simulink model "VehCtrlMdel240829_autosar"  (R2019b)
settings: Solver=FixedStepDiscrete  StartTime=0.0  StopTime=10.0  FixedStep=0.0005  RelTol=1e-3  EnableMultiTasking=on
values from neighbouring files (symbols this model uses):
  Ax_OffSet = 0.0    [VehCtrlMdelDictionary.sldd]    (also in VehPara.m = 0)
  Ay_OffSet = 0.0    [VehCtrlMdelDictionary.sldd]    (also in VehPara.m = 0)
  Caf = 460.0    [VehCtrlMdelDictionary.sldd]    (also in VehPara.m = 460; trqvparameter.m = 460)
  Car = 440.0    [VehCtrlMdelDictionary.sldd]    (also in VehPara.m = 440; trqvparameter.m = 440)
  dwf = 1.2    [VehCtrlMdelDictionary.sldd]    (also in VehPara.m; trqvparameter.m)
  Ki = 1.0    [VehCtrlMdelDictionary.sldd]    (also in VehPara.m = 1; trqvparameter.m = 1)
  Kp = 2.0    [VehCtrlMdelDictionary.sldd]    (also in VehPara.m = 2; trqvparameter.m = 2)
  Ldwf = 1.2    [VehCtrlMdelDictionary.sldd]    (also in VehPara.m)
  Ldwr = 1.16    [VehCtrlMdelDictionary.sldd]    (also in VehPara.m)
  lf = 0.761    [VehCtrlMdelDictionary.sldd]    (also in VehPara.m; trqvparameter.m)
  lr = 0.831    [VehCtrlMdelDictionary.sldd]    (also in VehPara.m; trqvparameter.m)
  m = 340.0    [VehCtrlMdelDictionary.sldd]    (also in VehPara.m = 340; trqvparameter.m = 340)
  Offset_Angle = 0.0    [VehCtrlMdelDictionary.sldd]    (also in VehPara.m = 0)
  Qa = 0.1    [VehCtrlMdelDictionary.sldd]    (also in VehPara.m)
  Ra = 2.0    [VehCtrlMdelDictionary.sldd]    (also in VehPara.m = 2)
  RearRatio = 0.8    [VehCtrlMdelDictionary.sldd]    (also in VehPara.m)
  Rt = 0.2    [VehCtrlMdelDictionary.sldd]    (also in VehPara.m; trqvparameter.m)
  thr1 = 2.0    [VehCtrlMdelDictionary.sldd]    (also in VehPara.m = 2)
  thr2 = 0.5    [VehCtrlMdelDictionary.sldd]    (also in VehPara.m)
  thr3 = 0.8    [VehCtrlMdelDictionary.sldd]    (also in VehPara.m)
  thr4 = 0.5    [VehCtrlMdelDictionary.sldd]    (also in VehPara.m)
  thr5 = -0.5    [VehCtrlMdelDictionary.sldd]    (also in VehPara.m)
  TrqRquRate = 0.1    [VehCtrlMdelDictionary.sldd]    (also in VehPara.m)
  YawRate_OffSet = 0.0    [VehCtrlMdelDictionary.sldd]    (also in VehPara.m = 0)
undefined symbols (not defined in the file or in its folder): DiscIntNeverNeededParam, I_AN07_5V, I_AN08_5V, I_AN10_5V, I_SW01_L, I_SW02_L, I_SW03_L, Iz, O_SW12_HS1A, O_SW14_HS1A, PWM3
libraries: simulink x126, ec5744lib x77, canmsglib x18
(part 5 of 5)

== stateflow chart VehCtrlMdel240829_autosar/Drive_Ready/Subsystem/Chart2 ==
  state VehStat [parallel]
    settings: executionOrder=1
    state WaitForEngine
      en:
      send(AMKCANOFF,AMKCANenable);
      send(AMKDCOFF,AMKDCon);
      send(MCDCEnableOFF,MCDCEnable);
      send(InverterOFF,MC_InverterOn);
    state Standby
    state Trans
    state Guard
    state InitStateBack
    state Ready
    state Init
      en:
      errorReset = 1;
    state MCUReadyFail
    WaitForEngine -> Standby : [aMCUReady&&bMCUReady&&cMCUReady]
    Standby -> Guard [order 2] : [KeyPressed&&Brk&&ACC_Release&&cMCUReady&&aMCUReady&&bMCUReady]
    Trans -> Ready : after(2.5,sec){send(EbeepOFF,BeeperStat)}
    Guard -> Trans [order 1] : after(0.25,sec){send(EbeepON,BeeperStat)}
    Guard -> Standby [order 2] : [~KeyPressed||~Brk||~ACC_Release]
    Standby -> WaitForEngine [order 1] : [~aMCUReady||~bMCUReady||~cMCUReady]
    Guard -> InitStateBack [order 3] : [~cMCUReady||~aMCUReady||~bMCUReady]
    Init -> WaitForEngine : [after(1,sec)]
    MCUReadyFail -> WaitForEngine
    InitStateBack -> WaitForEngine
    Ready -> InitStateBack [order 2] : [~HVCutOFF]
    (default) -> Init
    Ready -> MCUReadyFail [order 1] : [~cMCUReady||~aMCUReady||~bMCUReady]
  state BeeperStat [parallel]
    settings: executionOrder=2
    state OFF
    state ON
    (default) -> BeeperStat.OFF
    BeeperStat.OFF -> BeeperStat.ON : EbeepON
    BeeperStat.ON -> BeeperStat.OFF : EbeepOFF
  state AMKDCon [parallel]
    settings: executionOrder=6
    state OFF
    state ON
    (default) -> AMKDCon.OFF
    AMKDCon.OFF -> AMKDCon.ON : AMKDCON
    AMKDCon.ON -> AMKDCon.OFF : AMKDCOFF
  state MCDCEnable [parallel]
    settings: executionOrder=7
    state OFF
    state ON
    (default) -> MCDCEnable.OFF
    MCDCEnable.OFF -> MCDCEnable.ON : MCDCEnableON
    MCDCEnable.ON -> MCDCEnable.OFF : MCDCEnableOFF
  state AMKDCready [parallel]
    settings: executionOrder=4
    state start
    state AMKCAN
      en:
      send(AMKCANON,AMKCANenable);
    state MC_DCready
    state MCDCOncheck
    state DCOnCheckPass
    state MC_DCOnFail
      en:
      send(AMKDCOFF,AMKDCon);
      send(MCDCEnableOFF,MCDCEnable);
      send(InverterOFF,MC_InverterOn);
    state AMKDCOnFinish
    state SYSRDYCECK
    state MCDCEnableState
      en:
      send(MCDCEnableON,MCDCEnable);
    state MC_InverterOn_State
      en:
      send(InverterON,MC_InverterOn);
    (default) -> start
    AMKCAN -> MC_DCready : [SWAMKDCOn]
    MC_DCready -> MCDCOncheck [order 2] : after(0.1,sec){send(AMKDCON,AMKDCon)}
    MCDCOncheck -> DCOnCheckPass [order 1] : after(0.1,sec)
    start -> AMKCAN : after(10,sec)
    DCOnCheckPass -> MCDCEnableState : after(0.1,sec)[MCFLDCOncheck&&MCFRDCOncheck]
    MCDCOncheck -> MC_DCOnFail [order 2] : [~MCFRDCOncheck||~MCFLDCOncheck]
    MC_DCready -> AMKCAN [order 1] : [~SWAMKDCOn]
    SYSRDYCECK -> MC_DCOnFail [order 2] : [~MCFL_SYSREADY||~MCFR_SYSREADY]
    SYSRDYCECK -> AMKDCOnFinish [order 1] : [MCFL_SYSREADY&&MCFR_SYSREADY]
    MC_InverterOn_State -> SYSRDYCECK
    MCDCEnableState -> MC_InverterOn_State : after(0.1,sec)
  state Output [parallel]
    du:
    VehReady = in(VehStat.Ready);
    VehStandby = in(VehStat.Standby);
    BeeperStOut = in(BeeperStat.ON);
    AMKCANready = in(AMKCANenable.ON);
    MCFL_DCOn_setpoints = in(AMKDCon.ON);
    MCFR_DCOn_setpoints = in(AMKDCon.ON);
    MCFL_DCEnable = in(MCDCEnable.ON);
    MCFR_DCEnable = in(MCDCEnable.ON);
    MC_DCOnError = in(AMKDCready.MC_DCOnFail);
    MCFL_InverterOn = in(MC_InverterOn.ON);
    MCFR_InverterOn = in(MC_InverterOn.ON);
    settings: executionOrder=3
  state AMKCANenable [parallel]
    settings: executionOrder=5
    state OFF
    state ON
    (default) -> AMKCANenable.OFF
    AMKCANenable.OFF -> AMKCANenable.ON : AMKCANON
    AMKCANenable.ON -> AMKCANenable.OFF : AMKCANOFF
  state MC_InverterOn [parallel]
    settings: executionOrder=8
    state OFF
    state ON
    (default) -> MC_InverterOn.OFF
    MC_InverterOn.OFF -> MC_InverterOn.ON : InverterON
    MC_InverterOn.ON -> MC_InverterOn.OFF : InverterOFF
  data: Brk input boolean size=1; KeyPressed input boolean size=1; VehReady output boolean size=1; BeeperStOut output boolean size=1; VehStandby output boolean; ACC_Release input boolean; cMCUReady input; aMCUReady input; bMCUReady input; AMKCANready output; MCFL_DCOn_setpoints output; MCFRDCOncheck input; MCFLDCOncheck input; MCFR_DCOn_setpoints output; MCFR_DCEnable output; MCFR_InverterOn output; MC_DCOnError output; MCFL_InverterOn output; MCFL_DCEnable output; MCFL_SYSREADY input; MCFR_SYSREADY input; SWAMKDCOn input; HVCutOFF input; errorReset output
  events: EbeepON local FUNCTION_CALL_EVENT; EbeepOFF local FUNCTION_CALL_EVENT; AMKCANOFF local FUNCTION_CALL_EVENT; AMKCANON local FUNCTION_CALL_EVENT; AMKDCON local FUNCTION_CALL_EVENT; AMKDCOFF local FUNCTION_CALL_EVENT; InverterOFF local FUNCTION_CALL_EVENT; InverterON local FUNCTION_CALL_EVENT; MCDCEnableON local FUNCTION_CALL_EVENT; MCDCEnableOFF local FUNCTION_CALL_EVENT

== matlab function VehCtrlMdel240829_autosar/CTRL/MoTrqReq/DYC/Wtarget ==
  data: Vx input size=1; Wtarget output size=1; a input size=1; Car input size=1; Caf input size=1; lr input size=1; lf input size=1; m input; u input; btarget output
function [Wtarget,btarget] = fcn(Vx,a,Car,Caf,lr,lf,m,u)
Wdes = Vx*a/(lf+lr+(m*Vx*Vx*(lr*Car-lf*Caf)/Caf/Car/(lr+lf)/2));
% Wu = 0.85*u*9.8/Vx;
% if abs(Wdes)<=Wu
Wtarget = Wdes;
% else
%    Wtarget = Wu*sign(Wdes);
% end
bdes = (lr-lf*m*Vx*Vx/Car/(lf+lr)/2)*a/(lr+lf+m*Vx*Vx*(lr*Car-lf*Caf)/Car/Caf/(lf+lr)/2);
bu = atan(0.02*u*9.8);
if abs(bdes)<=bu
btarget = bdes;
else
    btarget = bu*sign(bdes);
end

== stateflow chart VehCtrlMdel240829_autosar/Input_Processing/Function-Call Subsystem/AccBrkPedal/Timer ==
  state Trigger
    en:
    x = x + 0.01;
    Exit=0;
  state Out
    en:
    Exit=1;
    x=0;
  state InterState
    en:
    x=0;
  Trigger -> Trigger [order 1] : [Trigger&&x<CountTime]
  Trigger -> Out [order 2] : [x>=CountTime]
  (default) -> Trigger
  Out -> Trigger : [~Trigger]
  InterState -> Trigger : [Trigger]
  Trigger -> InterState [order 3] : [x<CountTime&&~Trigger]
  data: Trigger input; CountTime input; Exit output; x local =0

== stateflow chart VehCtrlMdel240829_autosar/CTRL/MoTrqReq/DYC/Timer1 ==
  state Trigger
    en:
    x = x + 0.01;
    Exit=0;
  state Out
    en:
    Exit=1;
    x=0;
  state InterState
    en:
    x=0;
  Trigger -> Trigger [order 1] : [Trigger&&x<CountTime]
  Trigger -> Out [order 2] : [x>=CountTime]
  (default) -> Trigger
  Out -> Trigger : [~Trigger]
  InterState -> Trigger : [Trigger]
  Trigger -> InterState [order 3] : [x<CountTime&&~Trigger]
  data: Trigger input; CountTime input; Exit output; x local =0

== stateflow chart VehCtrlMdel240829_autosar/CTRL/PwrTrainTempPrtct/Timer1 ==
  state Trigger
    en:
    x = x + 0.01;
    Exit=0;
  state Out
    en:
    Exit=1;
    x=0;
  state InterState
    en:
    x=0;
  Trigger -> Trigger [order 1] : [Trigger&&x<CountTime]
  Trigger -> Out [order 2] : [x>=CountTime]
  (default) -> Trigger
  Out -> Trigger : [~Trigger]
  InterState -> Trigger : [Trigger]
  Trigger -> InterState [order 3] : [x<CountTime&&~Trigger]
  data: Trigger input; CountTime input; Exit output; x local =0

== stateflow chart VehCtrlMdel240829_autosar/CTRL/PwrTrainTempPrtct/Timer2 ==
  state Trigger
    en:
    x = x + 0.01;
    Exit=0;
  state Out
    en:
    Exit=1;
    x=0;
  state InterState
    en:
    x=0;
  Trigger -> Trigger [order 1] : [Trigger&&x<CountTime]
  Trigger -> Out [order 2] : [x>=CountTime]
  (default) -> Trigger
  Out -> Trigger : [~Trigger]
  InterState -> Trigger : [Trigger]
  Trigger -> InterState [order 3] : [x<CountTime&&~Trigger]
  data: Trigger input; CountTime input; Exit output; x local =0

== stateflow chart VehCtrlMdel240829_autosar/CTRL/MoTrqReq/Chart ==
  state A
    en:
    if abs(IMU_Ay)>0.5
    a=atan(IMU_Ax/IMU_Ay)*180/pi;
    else
    a = 0;
    end
    b=sqrt(power(IMU_Ax,2)+power(IMU_Ay,2));
  state InitState
  state DYC_Disenable
    en:
    DYC_Enable_OUT=0;
    DYC_flag=0;
  state TCSR_Disenable
    en:
    TCSR_Enable_OUT=0;
  state TCSR_Enable
    en:
    TCSR_Enable_OUT=1;
  state TCSF_Disenable
    en:
    TCSF_Enable_OUT=0;
  state TCSF_Enable
    en:
    TCSF_Enable_OUT=1;
  state DYC_Enable
    en:
    DYC_Enable_OUT=1;
    DYC_flag=1;
  state B
    en:
    TCSR_Enable_OUT=1;
  state F_TVD_TCS_STATE
  state C
    en:
    TCSR_Enable_OUT=0;
  (default) -> InitState [order 1]
  (default) -> A [order 2]
  A -> A
  InitState -> TCSR_Disenable [order 5] : [~TCSR_Enable]
  InitState -> TCSR_Enable [order 6] : [TCSR_Enable]
  TCSF_Disenable -> InitState : [TCSF_Enable]
  InitState -> TCSF_Disenable [order 4] : [~TCSF_Enable]
  InitState -> TCSF_Enable [order 3] : [TCSF_Enable&&DYC_flag&&~DYC_flag&&a>60&&a<-60&&IMU_Ax>2&&b<5&&IMU_Yaw<50]
  TCSF_Enable -> InitState : [b>5]
  DYC_Disenable -> InitState : [DYC_Enable]
  InitState -> DYC_Disenable [order 2] : [~DYC_Enable]
  DYC_Enable -> InitState : [IMU_Yaw>=50||IMU_Ay>=5||b>=5]
  InitState -> DYC_Enable [order 1] : [DYC_Enable&&IMU_Yaw<=50&&IMU_Ay<5&&b<5]
  TCSR_Disenable -> TCSR_Enable : [TCSR_Enable]
  TCSR_Enable -> TCSR_Disenable : [~TCSR_Enable]
  F_TVD_TCS_STATE -> B [order 1] : [DYC_flag&&IMU_Yaw<=30&&a>=30&&a<=-30&&b<=3]
  B -> F_TVD_TCS_STATE : [~DYC_flag||IMU_Yaw>30||a>30||a>-30||b>3]
  (default) -> F_TVD_TCS_STATE [order 3]
  C -> F_TVD_TCS_STATE : [DYC_flag&&IMU_Yaw<=30&&a>=30&&a<=-30&&b<=3]
  F_TVD_TCS_STATE -> C [order 2] : [~DYC_flag||IMU_Yaw>30||a>30||a>-30||b>3]
  data: DYC_Enable input; TCSF_Enable input; TCSR_Enable input; TCSFR_flgActv input; TCSFL_flgActv input; TCSR_flgActv input; TVD_Trigger input; DYC_Enable_OUT output; TCSR_Enable_OUT output; TCSF_Enable_OUT output; IMU_Ax input; IMU_Ay input; IMU_Yaw input; a local; b local; DYC_flag local

== stateflow chart VehCtrlMdel240829_autosar/Input_Processing/Function-Call Subsystem/SWAS/Timer ==
  state Trigger
    en:
    x = x + 0.01;
    Exit=0;
  state Out
    en:
    Exit=1;
    x=0;
  state InterState
    en:
    x=0;
  Trigger -> Trigger [order 1] : [Trigger&&x<CountTime]
  Trigger -> Out [order 2] : [x>=CountTime]
  (default) -> Trigger
  Out -> Trigger : [~Trigger]
  InterState -> Trigger : [Trigger]
  Trigger -> InterState [order 3] : [x<CountTime&&~Trigger]
  data: Trigger input; CountTime input; Exit output; x local =0

== stateflow chart VehCtrlMdel240829_autosar/Input_Processing/Function-Call Subsystem/WhlSpdii_mps/Timer ==
  state Trigger
    en:
    x = x + 0.01;
    Exit=0;
  state Out
    en:
    Exit=1;
    x=0;
  state InterState
    en:
    x=0;
  Trigger -> Trigger [order 1] : [Trigger&&x<CountTime]
  Trigger -> Out [order 2] : [x>=CountTime]
  (default) -> Trigger
  Out -> Trigger : [~Trigger]
  InterState -> Trigger : [Trigger]
  Trigger -> InterState [order 3] : [x<CountTime&&~Trigger]
  data: Trigger input; CountTime input; Exit output; x local =0

== stateflow chart VehCtrlMdel240829_autosar/Input_Processing/Function-Call Subsystem/WhlSpdii_mps/Timer1 ==
  state Trigger
    en:
    x = x + 0.01;
    Exit=0;
  state Out
    en:
    Exit=1;
    x=0;
  state InterState
    en:
    x=0;
  Trigger -> Trigger [order 1] : [Trigger&&x<CountTime]
  Trigger -> Out [order 2] : [x>=CountTime]
  (default) -> Trigger
  Out -> Trigger : [~Trigger]
  InterState -> Trigger : [Trigger]
  Trigger -> InterState [order 3] : [x<CountTime&&~Trigger]
  data: Trigger input; CountTime input; Exit output; x local =0

== stateflow chart VehCtrlMdel240829_autosar/Input_Processing/Function-Call Subsystem/WhlSpdii_mps/Timer2 ==
  state Trigger
    en:
    x = x + 0.01;
    Exit=0;
  state Out
    en:
    Exit=1;
    x=0;
  state InterState
    en:
    x=0;
  Trigger -> Trigger [order 1] : [Trigger&&x<CountTime]
  Trigger -> Out [order 2] : [x>=CountTime]
  (default) -> Trigger
  Out -> Trigger : [~Trigger]
  InterState -> Trigger : [Trigger]
  Trigger -> InterState [order 3] : [x<CountTime&&~Trigger]
  data: Trigger input; CountTime input; Exit output; x local =0

== stateflow chart VehCtrlMdel240829_autosar/Input_Processing/Function-Call Subsystem/WhlSpdii_mps/Timer3 ==
  state Trigger
    en:
    x = x + 0.01;
    Exit=0;
  state Out
    en:
    Exit=1;
    x=0;
  state InterState
    en:
    x=0;
  Trigger -> Trigger [order 1] : [Trigger&&x<CountTime]
  Trigger -> Out [order 2] : [x>=CountTime]
  (default) -> Trigger
  Out -> Trigger : [~Trigger]
  InterState -> Trigger : [Trigger]
  Trigger -> InterState [order 3] : [x<CountTime&&~Trigger]
  data: Trigger input; CountTime input; Exit output; x local =0

== matlab function VehCtrlMdel240829_autosar/CTRL/MoTrqReq/DYC/MATLAB Function ==
  data: WSA input; Mz output; WSAV input; lf input; lr input; Caf input; Car input; Iz input; m input; Vx input
function Mz = fcn(WSA,WSAV,lf,lr,Caf,Car,Iz,m,Vx)

Mz = (((lf*lf*Caf+lr*lr*Car)/Iz/Vx)*(-Caf/m/Vx)-((lf*Caf-lr*Car)/m/Vx/Vx-1)*(-lf*Caf/Iz))*Iz*WSA/((lf*Caf-lr*Car)/m/Vx/Vx-1)-(-Caf/m/Vx)*Iz*WSAV/((lf*Caf-lr*Car)/m/Vx/Vx-1);

== stateflow chart VehCtrlMdel240829_autosar/Input_Processing/Subsystem/WhlSlpageJudgment/Timer ==
  state Trigger
    en:
    x = x + 0.01;
    Exit=0;
  state Out
    en:
    Exit=1;
    x=0;
  state InterState
    en:
    x=0;
  Trigger -> Trigger [order 1] : [Trigger&&x<CountTime]
  Trigger -> Out [order 2] : [x>=CountTime]
  (default) -> Trigger
  Out -> Trigger : [~Trigger]
  InterState -> Trigger : [Trigger]
  Trigger -> InterState [order 3] : [x<CountTime&&~Trigger]
  data: Trigger input; CountTime input; Exit output; x local =0

== stateflow chart VehCtrlMdel240829_autosar/Input_Processing/Subsystem/WhlSpdSelect/Timer1 ==
  state Trigger
    en:
    x = x + 0.01;
    Exit=0;
  state Out
    en:
    Exit=1;
    x=0;
  state InterState
    en:
    x=0;
  Trigger -> Trigger [order 1] : [Trigger&&x<CountTime]
  Trigger -> Out [order 2] : [x>=CountTime]
  (default) -> Trigger
  Out -> Trigger : [~Trigger]
  InterState -> Trigger : [Trigger]
  Trigger -> InterState [order 3] : [x<CountTime&&~Trigger]
  data: Trigger input; CountTime input; Exit output; x local =0

== stateflow chart VehCtrlMdel240829_autosar/Input_Processing/Subsystem/WhlSpdSelect/Timer2 ==
  state Trigger
    en:
    x = x + 0.01;
    Exit=0;
  state Out
    en:
    Exit=1;
    x=0;
  state InterState
    en:
    x=0;
  Trigger -> Trigger [order 1] : [Trigger&&x<CountTime]
  Trigger -> Out [order 2] : [x>=CountTime]
  (default) -> Trigger
  Out -> Trigger : [~Trigger]
  InterState -> Trigger : [Trigger]
  Trigger -> InterState [order 3] : [x<CountTime&&~Trigger]
  data: Trigger input; CountTime input; Exit output; x local =0

== stateflow chart VehCtrlMdel240829_autosar/Input_Processing/Subsystem/WhlSlpageJudgment/Timer1 ==
  state Trigger
    en:
    x = x + 0.01;
    Exit=0;
  state Out
    en:
    Exit=1;
    x=0;
  state InterState
    en:
    x=0;
  Trigger -> Trigger [order 1] : [Trigger&&x<CountTime]
  Trigger -> Out [order 2] : [x>=CountTime]
  (default) -> Trigger
  Out -> Trigger : [~Trigger]
  InterState -> Trigger : [Trigger]
  Trigger -> InterState [order 3] : [x<CountTime&&~Trigger]
  data: Trigger input; CountTime input; Exit output; x local =0

== stateflow chart VehCtrlMdel240829_autosar/Input_Processing/Subsystem/WhlSlpageJudgment/Timer2 ==
  state Trigger
    en:
    x = x + 0.01;
    Exit=0;
  state Out
    en:
    Exit=1;
    x=0;
  state InterState
    en:
    x=0;
  Trigger -> Trigger [order 1] : [Trigger&&x<CountTime]
  Trigger -> Out [order 2] : [x>=CountTime]
  (default) -> Trigger
  Out -> Trigger : [~Trigger]
  InterState -> Trigger : [Trigger]
  Trigger -> InterState [order 3] : [x<CountTime&&~Trigger]
  data: Trigger input; CountTime input; Exit output; x local =0

== stateflow chart VehCtrlMdel240829_autosar/Input_Processing/Subsystem/WhlSlpageJudgment/Timer3 ==
  state Trigger
    en:
    x = x + 0.01;
    Exit=0;
  state Out
    en:
    Exit=1;
    x=0;
  state InterState
    en:
    x=0;
  Trigger -> Trigger [order 1] : [Trigger&&x<CountTime]
  Trigger -> Out [order 2] : [x>=CountTime]
  (default) -> Trigger
  Out -> Trigger : [~Trigger]
  InterState -> Trigger : [Trigger]
  Trigger -> InterState [order 3] : [x<CountTime&&~Trigger]
  data: Trigger input; CountTime input; Exit output; x local =0
